simulink model "r2_deng_tvg_2013a"  (R2013a)
(part 3 of 43)

  edge_detect2/1(out) -> [mrst]  "mrst"
  edge_detect1/1(out) -> [msync]  "msync"
  edge_detect4/1(out) -> [clr_status]  "clr_status"
  Counter Free-Running/1 -> Relational Operator1/2, Relational Operator/2
  Constant1/1 -> Relational Operator/1
  Constant/1 -> Relational Operator1/1
  [local_time] -> slice1/1, slice2/1
  edge_detect3/1(out) -> [up_cnt_rst]  "mrst"
  Constant28/1 -> control/3(sim_3)
  Constant44/1 -> control/1(sim_1)
  Constant24/1 -> control/2(sim_2)
  Constant33/1 -> control/6(sim_6)
  Constant30/1 -> control/5(sim_5)
  Constant36/1 -> control/4(sim_4)
  Relational Operator/1 -> control/8(sim_8)
  Relational Operator1/1 -> control/7(sim_7)
  [tick_offset] -> ticks_since_mrst/3(offset)
  edge_detect10/1(out) -> [load_tick_offset]  "mrst"
  Constant20/1 -> control/9(sim_9)
  digitiser_id/1(in_digitiser_serial) -> bus_create/1(in1)
  digitiser_id/2(in_digitiser_type) -> bus_create/2(in2)
  Constant43/1 -> flag_setup/3(sim_3)
  Constant42/1 -> flag_setup/2(sim_2)
  Constant39/1 -> flag_setup/1(sim_1)
  Counter Free-Running3/1 -> Relational Operator4/2
  Constant48/1 -> Relational Operator4/1
  Relational Operator4/1 -> flag_setup/4(sim_4)
  Constant52/1 -> start_flag_msw/1(sim_1)
  Constant53/1 -> start_flag_lsw/1(sim_1)
  Constant51/1 -> end_flag_msw/1(sim_1)
  Constant50/1 -> end_flag_lsw/1(sim_1)
  Concat4/1 -> Delay49/1  "starttime"
  Concat5/1 -> Delay50/1  "stoptime"
  [flag_start_time] -> Delay46/1
  [local_time] -> Delay45/1, Delay47/1
  [flag_end_time] -> Delay48/1, Delay51/1
  Relational/1 -> Logical2/2  "start_okay"
  [flag_armed] -> Delay44/1
  Relational1/1 -> Logical4/2  "end_okay"
  Logical2/1 -> Delay23/1  "start_okay"
  Logical4/1 -> Logical3/1  "end_okay"
  edge_detect9/1(out) -> [load_flag_time]  "loadtimes"
  Constant4/1 -> Register1/1
  edge_detect8/1(out) -> [reset_flag_time]  "rst"
  [reset_flag_time] -> Register1/2
  [load_flag_time] -> Register1/3
  Register1/1 -> [flag_armed]  "armed"
  Relational Operator3/1 -> flag_setup/5(sim_5)
  Relational2/1 -> Delay22/1  "zero_stop"
  Constant2/1 -> Relational2/2
  Logical3/1 -> Logical1/2  "eokay"
  Counter Free-Running2/1 -> Relational Operator3/2
  Constant5/1 -> Relational Operator3/1
  Logical5/1 -> sample_masking/2(den_in)
  Constant49/1 -> start_time_msw/1(sim_1)
  Constant54/1 -> start_time_lsw/1(sim_1)
  Constant3/1 -> end_time_msw/1(sim_1)
  Constant11/1 -> end_time_lsw/1(sim_1)
  Relational3/1 -> Logical6/2  "start_okay"
  Relational4/1 -> Logical8/2  "end_okay"
  [start_time] -> Delay39/1
  Relational6/1 -> Delay15/1  "first_sample"
  [end_time] -> Delay41/1
  Relational7/1 -> Delay16/1  "last_sample"
  [sample_end] -> sample_masking/6(sample_end)
  [sample_start] -> sample_masking/5(sample_start)
  sample_masking/2(den_out) -> Delay126/1  "enable"
  sample_masking/3(data_mask) -> Delay127/1  "mask"
  edge_detect11/1(out) -> [reset_en_time]  "reset_en_time"
  Relational Operator5/1 -> control_output/2(sim_2)
  Counter Free-Running4/1 -> Relational Operator6/2, Relational Operator5/2
  Constant38/1 -> Relational Operator5/1
  edge_detect12/1(out) -> [load_en_time]  "load_en_time"
  Concat/1 -> Delay42/1
  Concat1/1 -> Delay43/1
  Constant22/1 -> Register2/1
  [reset_en_time] -> Register2/2
  [load_en_time] -> Register2/3
  Register2/1 -> [en_armed]  "armed"
  Logical6/1 -> Delay17/1  "start_okay"
  Logical8/1 -> Logical7/1  "end_okay"
  Logical7/1 -> Logical5/2
  Constant34/1 -> Delay37/1
  Relational5/1 -> Delay14/1
  Constant29/1 -> control_output/3(sim_3)
  Constant47/1 -> control_output/4(sim_4)
  Constant31/1 -> Relational Operator6/1
  Relational Operator6/1 -> control_output/1(sim_1)
  [data_enable] -> Delay129/1
  [sample_mask] -> Delay130/1
  Constant23/1 -> Mux3/2
  [adc_count] -> Concat3/1
  [adc_flag] -> Concat3/3
  [ndiode_flag] -> Concat3/4
  Constant55/1 -> Concat3/2
  Concat3/1 -> Mux3/3
  [flag_en] -> Mux3/1
  Constant46/1 -> tick_offset_msw/1(sim_1)
  Constant7/1 -> tick_offset_lsw/1(sim_1)
  Concat2/1 -> Register3/1
  [load_tick_offset] -> Register3/2
  Register3/1 -> [tick_offset]
  Delay1/1 -> [status0]
  fifo2/1(fifo_data80) -> pipeline104/1(d)  "data00"
  fifo2/2(fifo_dv) -> pipeline105/1(d)  "dv00"
  fifo2/3(word_start) -> pipeline106/1(d)  "ws00"
  fifo2/4(pkt_start) -> pipeline107/1(d)  "ps00"
  fifo2/5(fifo_full) -> Terminator3/1  "full00"
  fifo2/6(fifo_empty) -> Terminator6/1  "empty00"
  fifo3/1(fifo_data80) -> pipeline108/1(d)  "data01"
  fifo3/2(fifo_dv) -> pipeline109/1(d)  "dv01"
  fifo3/3(word_start) -> pipeline110/1(d)  "ws01"
  fifo3/4(pkt_start) -> pipeline111/1(d)  "ps01"
  pack_80_64_2/3(data64) -> pipeline123/1(d)  "d64_00"
  pack_80_64_2/2(valid64) -> pipeline122/1(d)  "v64_01"
  pack_80_64_2/1(ready64) -> pipeline121/1(d)  "r64_01"
  fifo3/5(fifo_full) -> Terminator4/1
  fifo3/6(fifo_empty) -> Terminator5/1
  [hdr_0x3101] -> bus_create3/1(in1)
  [pol1_id] -> bus_create3/2(in2)
  [hdr_0x3101] -> bus_create2/1(in1)
  [pol1_id] -> bus_create2/2(in2)
  [speadtime0] -> spead_pack2/4(hdr_heap_id), spead_pack2/8(hdr5_0x1600_DIR)  "timein0"
  bus_create3/1(bus_out) -> spead_pack2/9(hdr6_0x3101_DIR)
  [status2] -> spead_pack2/10(hdr7_0x3102_DIR)
  bus_create2/1(bus_out) -> spead_pack3/9(hdr6_0x3101_DIR)
  [status3] -> spead_pack3/10(hdr7_0x3102_DIR)
  [speadtime1] -> spead_pack3/8(hdr5_0x1600_DIR), spead_pack3/4(hdr_heap_id)  "timein1"
  pack_80_64_1/1(ready64) -> pipeline118/1(d)  "r64_00"
  pack_80_64_1/2(valid64) -> pipeline119/1(d)  "v64_00"
  pack_80_64_1/3(data64) -> pipeline120/1(d)  "d64_00"
  [spead_heapsize] -> spead_pack2/5(hdr_heap_size)
  [spead_heapoffset] -> spead_pack2/6(hdr_heap_offset)
  [spead_pktlen] -> spead_pack2/7(hdr_pkt_len_words)
  [spead_heapsize] -> spead_pack3/5(hdr_heap_size)
  [spead_heapoffset] -> spead_pack3/6(hdr_heap_offset)
  [spead_pktlen] -> spead_pack3/7(hdr_pkt_len_words)
  spead_pack3/4(data_overflow) -> Terminator2/1
  [adc_data_offset] -> spead_pack2/11(hdr8_0x3300)
  [adc_data_offset] -> spead_pack3/11(hdr8_0x3300)
  spead_pack2/4(data_overflow) -> Terminator1/1
  spead_pack2/3(eof) -> pipeline62/1(d)
  spead_pack2/1(data_out) -> pipeline60/1(d)  "packd"
  spead_pack2/2(valid_out) -> pipeline61/1(d)  "packv"
  spead_pack3/1(data_out) -> pipeline63/1(d)
  spead_pack3/2(valid_out) -> pipeline64/1(d)
  spead_pack3/3(eof) -> pipeline65/1(d)
  Inverter1/1 -> fifo3/2(fifo_we_en)
  [tvg_select1] -> Delay106/1
  Mux1/1 -> Assert1/1  "d80_0"
  [data_80_1] -> Delay109/1
  [tvg_pol1] -> Delay108/1
  Assert1/1 -> fifo3/1(data80), fifo2/1(data80)
  [fifoselect] -> Inverter1/1, fifo2/2(fifo_we_en)
  [gbe_txen] -> Logical13/1, Logical10/2
  Logical10/1 -> pipeline86/1(d)
  [gbe_port0] -> gbe0/5(tx_dest_port)
  Constant56/1 -> gbe0/8(rx_overrun_ack), gbe0/7(rx_ack)
  [spead_valid0] -> Logical10/1
  pipeline83/1(q) -> gbe0/2(tx_data)
  [gbe_ip0] -> gbe0/4(tx_dest_ip)
  [gbe_rst] -> pipeline68/1(d)
  [gbe_txen] -> Logical14/1, Logical9/2
  Logical9/1 -> pipeline85/1(d)
  [gbe_port1] -> gbe1/5(tx_dest_port)
  Constant18/1 -> gbe1/8(rx_overrun_ack), gbe1/7(rx_ack)
  [spead_valid1] -> Logical9/1
  pipeline80/1(q) -> gbe1/2(tx_data)
  [gbe_ip1] -> gbe1/4(tx_dest_ip)
  [gbe_rst] -> pipeline70/1(d)
  [gbe_txen] -> Logical15/1, Logical12/2
  Logical12/1 -> pipeline82/1(d)
  [gbe_port2] -> gbe2/5(tx_dest_port)
  Constant25/1 -> gbe2/8(rx_overrun_ack), gbe2/7(rx_ack)
  [spead_valid2] -> Logical12/1
  pipeline77/1(q) -> gbe2/2(tx_data)
  [gbe_ip2] -> gbe2/4(tx_dest_ip)
  [gbe_txen] -> Logical16/1, Logical11/2
  Logical11/1 -> pipeline75/1(d)
  [gbe_port3] -> gbe3/5(tx_dest_port)
  Constant21/1 -> gbe3/8(rx_overrun_ack), gbe3/7(rx_ack)
  [spead_data3] -> pipeline74/1(d)
  [gbe_ip3] -> gbe3/4(tx_dest_ip)
  [clr_status] -> pipeline69/1(d)
  [clr_status] -> pipeline71/1(d)
  [spead_eof0] -> Logical13/2
  [spead_eof1] -> Logical14/2
  Logical15/1 -> pipeline87/1(d)
  [spead_eof2] -> Logical15/2
  Logical16/1 -> pipeline76/1(d)
  [spead_eof3] -> Logical16/2
  gbe0/1(led_up) -> Terminator77/1
  gbe0/2(led_rx) -> Terminator67/1
  gbe0/3(led_tx) -> Terminator72/1
  gbe0/4(tx_afull) -> Terminator73/1
  gbe0/5(tx_overflow) -> Terminator75/1
  gbe0/6(rx_data) -> Terminator66/1
  gbe0/7(rx_valid) -> Terminator68/1
  gbe0/8(rx_source_ip) -> Terminator69/1
  gbe0/9(rx_source_port) -> Terminator70/1
  gbe0/10(rx_end_of_frame) -> Terminator71/1
  gbe0/11(rx_bad_frame) -> Terminator74/1
  gbe0/12(rx_overrun) -> Terminator76/1
  gbe1/1(led_up) -> Terminator13/1
  gbe1/2(led_rx) -> Terminator8/1
  gbe1/3(led_tx) -> Terminator40/1
  gbe1/4(tx_afull) -> Terminator43/1
  gbe1/5(tx_overflow) -> Terminator10/1
  gbe1/6(rx_data) -> Terminator7/1
  gbe1/7(rx_valid) -> Terminator9/1
  gbe1/8(rx_source_ip) -> Terminator34/1
  gbe1/9(rx_source_port) -> Terminator37/1
  gbe1/10(rx_end_of_frame) -> Terminator38/1
  gbe1/11(rx_bad_frame) -> Terminator46/1
  gbe1/12(rx_overrun) -> Terminator11/1
  gbe2/1(led_up) -> Terminator21/1
  gbe2/2(led_rx) -> Terminator22/1
  gbe2/3(led_tx) -> Terminator28/1
  gbe2/4(tx_afull) -> Terminator29/1
  gbe2/5(tx_overflow) -> Terminator17/1
  gbe2/6(rx_data) -> Terminator14/1
  gbe2/7(rx_valid) -> Terminator24/1
  gbe2/8(rx_source_ip) -> Terminator25/1
  gbe2/9(rx_source_port) -> Terminator26/1
  gbe2/10(rx_end_of_frame) -> Terminator27/1
  gbe2/11(rx_bad_frame) -> Terminator30/1
  gbe2/12(rx_overrun) -> Terminator19/1
  gbe3/1(led_up) -> Terminator35/1
  gbe3/2(led_rx) -> Terminator36/1
  gbe3/3(led_tx) -> Terminator45/1
  gbe3/4(tx_afull) -> Terminator47/1
  gbe3/5(tx_overflow) -> Terminator32/1
  gbe3/6(rx_data) -> Terminator31/1
  gbe3/7(rx_valid) -> Terminator39/1
  gbe3/8(rx_source_ip) -> Terminator41/1
  gbe3/9(rx_source_port) -> Terminator42/1
  gbe3/10(rx_end_of_frame) -> Terminator44/1
  gbe3/11(rx_bad_frame) -> Terminator48/1
  gbe3/12(rx_overrun) -> Terminator33/1
  Logical13/1 -> pipeline84/1(d)
  Logical14/1 -> pipeline81/1(d)
  [spead_data0] -> pipeline83/1(d)
  [spead_data1] -> pipeline80/1(d)
  [spead_data2] -> pipeline77/1(d)
  [spead_valid3] -> Logical11/1
  scale_wng0/1(in_reg) -> pipeline41/1(d)
  scale_wng1/1(in_reg) -> pipeline43/1(d)
  scale_wng_corr/1(in_reg) -> pipeline42/1(d)
  wng0/1(bus_out) -> pipeline78/1(d)
  wng1/1(bus_out) -> pipeline89/1(d)
  cwg0/1(bus_out) -> pipeline90/1(d)
  cwg_corr/1(bus_out) -> pipeline92/1(d), pipeline91/1(d)
  cwg1/1(bus_out) -> pipeline93/1(d)
  bus_addsub/1(dout) -> Delay105/1
  bus_addsub2/1(dout) -> Delay6/1
  bus_addsub3/1(dout) -> Delay9/1
  bus_addsub1/1(dout) -> Delay5/1
  bus_addsub4/1(dout) -> pipeline50/1(d)
  bus_mult/1(a*b) -> Scope4/3, bus_convert/1(din)
  bus_addsub5/1(dout) -> pipeline53/1(d)
  scale_out0/1(in_reg) -> pipeline51/1(d)
  scale_out1/1(in_reg) -> pipeline52/1(d)
  Constant35/1 -> scale_wng0/1(sim_1)
  Constant37/1 -> scale_wng1/1(sim_1)
  Constant57/1 -> scale_wng_corr/1(sim_1)
  Constant58/1 -> scale_cwg0/1(sim_1)
  scale_cwg0/1(in_reg) -> pipeline44/1(d)
  freq_cwg0/1(in_reg) -> pipeline45/1(d)
  Constant59/1 -> freq_cwg0/1(sim_1)
  Constant64/1 -> scale_out0/1(sim_1)
  Constant65/1 -> scale_out1/1(sim_1)
  Constant60/1 -> scale_cwg1/1(sim_1)
  scale_cwg1/1(in_reg) -> pipeline48/1(d)
  freq_cwg1/1(in_reg) -> pipeline49/1(d)
  Constant61/1 -> freq_cwg1/1(sim_1)
  Constant62/1 -> scale_cwg_corr/1(sim_1)
  scale_cwg_corr/1(in_reg) -> pipeline46/1(d)
  Constant63/1 -> freq_cwg_corr/1(sim_1)
  pipeline21/1(q) -> edge_detect12/1(in)
  pipeline22/1(q) -> edge_detect11/1(in)
  pipeline23/1(q) -> [sample_start]
  pipeline24/1(q) -> [sample_end]
  Delay42/1 -> [start_time]
  Delay43/1 -> [end_time]
  Delay49/1 -> [flag_start_time]
  Delay50/1 -> [flag_end_time]
  pipeline41/1(q) -> wng0/1(scale_16_14)
  pipeline42/1(q) -> wng_corr/1(scale_16_14)
  pipeline43/1(q) -> wng1/1(scale_16_14)
  pipeline44/1(q) -> cwg0/1(freq)
  pipeline45/1(q) -> cwg0/2(scale)
  pipeline46/1(q) -> cwg_corr/1(freq)
  pipeline48/1(q) -> cwg1/1(freq)
  pipeline49/1(q) -> cwg1/2(scale)
  pipeline10/1(q) -> [gbe_ip3]
  pipeline11/1(q) -> [gbe_ip2]
  pipeline13/1(q) -> [gbe_ip0]
  pipeline9/1(q) -> [gbe_port0]
  Delay102/1 -> Mux/1
  Delay103/1 -> Mux/2
  Delay104/1 -> Mux/3
  Delay106/1 -> Mux1/1
  Delay126/1 -> [data_enable]
  Delay127/1 -> [sample_mask]
  Delay128/1 -> tvg_spead_time_with_pkt_ctr/1(localtime64)
  Delay129/1 -> tvg_spead_time_with_pkt_ctr/2(data_enable)
  Delay130/1 -> tvg_spead_time_with_pkt_ctr/3(data_mask)
  Delay131/1 -> [tvg_ltime]
  Delay132/1 -> [tvg_stime]
  Delay133/1 -> [tvg_pol0]
  Delay134/1 -> [tvg_pol1]
  [tvg_pol0] -> Delay103/1
  [data_80_0] -> Delay104/1
  Delay109/1 -> Mux1/3
  Delay108/1 -> Mux1/2
  Delay105/1 -> Delay139/1
  Delay5/1 -> Delay7/1
  Delay6/1 -> Delay2/1
  Delay9/1 -> Delay8/1
  Delay139/1 -> Scope4/2, bus_addsub4/1(a)
  Delay7/1 -> bus_addsub5/1(a)
  Delay8/1 -> bus_addsub5/2(b), Scope3/1
  pipeline25/1(q) -> Concat/1
  pipeline26/1(q) -> Concat/2
  pipeline27/1(q) -> Concat1/1
  pipeline28/1(q) -> Concat1/2
  pipeline29/1(q) -> [hdr_0x3101]
  pipeline30/1(q) -> [pol0_id]
  pipeline31/1(q) -> [pol1_id]
  control/1(in_up_cnt_rst) -> pipeline/1(d)
  pipeline/1(q) -> edge_detect3/1(in)
  control/2(in_tvg_select0) -> pipeline1/1(d)
  control/3(in_tvg_select1) -> pipeline2/1(d)
  control/4(in_clr_status) -> pipeline3/1(d)
  control/5(in_gbe_rst) -> pipeline4/1(d)
  control/6(in_gbe_txen) -> pipeline5/1(d)
  control/7(in_msync) -> pipeline6/1(d)
  control/8(in_mrst) -> pipeline7/1(d)
  control/9(in_load_tick_offset) -> pipeline8/1(d)
  pipeline8/1(q) -> edge_detect10/1(in)
  pipeline7/1(q) -> edge_detect2/1(in)
  pipeline6/1(q) -> edge_detect1/1(in)
  pipeline5/1(q) -> [gbe_txen]
  pipeline4/1(q) -> [gbe_rst]
  pipeline3/1(q) -> edge_detect4/1(in)
  pipeline2/1(q) -> [tvg_select1]
  pipeline1/1(q) -> [tvg_select0]
  pipeline12/1(q) -> [gbe_ip1]
  pipeline16/1(q) -> pipeline124/1(d), pipeline125/1(d)
  pipeline14/1(q) -> [gbe_port1]
  gbe_iptx0/1(in_reg) -> pipeline13/1(d)
  gbe_iptx1/1(in_reg) -> pipeline12/1(d)
  gbe_iptx2/1(in_reg) -> pipeline11/1(d)
  gbe_iptx3/1(in_reg) -> pipeline10/1(d)
  tick_offset_msw/1(in_reg) -> pipeline17/1(d)
  pipeline17/1(q) -> Concat2/1
  tick_offset_lsw/1(in_reg) -> pipeline18/1(d)
  pipeline18/1(q) -> Concat2/2
  slice1/1 -> pipeline20/1(d)
  pipeline20/1(q) -> local_time_lsw/1(out_reg)
  slice2/1 -> pipeline19/1(d)
  pipeline19/1(q) -> local_time_msw/1(out_reg)
  end_time_lsw/1(in_reg) -> pipeline28/1(d)
  end_time_msw/1(in_reg) -> pipeline27/1(d)
  start_time_lsw/1(in_reg) -> pipeline26/1(d)
  start_time_msw/1(in_reg) -> pipeline25/1(d)
  control_output/4(in_sample_end) -> pipeline24/1(d)
  control_output/3(in_sample_start) -> pipeline23/1(d)
  control_output/2(in_reset_en_time) -> pipeline22/1(d)
  control_output/1(in_load_en_time) -> pipeline21/1(d)
  bus_create/1(bus_out) -> pipeline29/1(d)
  receptor_id/2(in_pol0_id) -> pipeline30/1(d)
  receptor_id/3(in_pol1_id) -> pipeline31/1(d)
  flag_setup/1(in_adc_count) -> pipeline32/1(d)
  flag_setup/2(in_adc_flag) -> pipeline33/1(d)
  flag_setup/3(in_ndiode_flag) -> pipeline34/1(d)
  flag_setup/4(in_load_flags) -> pipeline35/1(d)
  flag_setup/5(in_reset_flags) -> pipeline36/1(d)
  pipeline36/1(q) -> edge_detect8/1(in)
  pipeline35/1(q) -> edge_detect9/1(in)
  pipeline34/1(q) -> [ndiode_flag]
  pipeline33/1(q) -> [adc_flag]
  pipeline32/1(q) -> [adc_count]
  start_flag_msw/1(in_reg) -> pipeline37/1(d)
  pipeline37/1(q) -> Concat4/1
  start_flag_lsw/1(in_reg) -> pipeline38/1(d)
  pipeline38/1(q) -> Concat4/2
  end_flag_msw/1(in_reg) -> pipeline39/1(d)
  pipeline39/1(q) -> Concat5/1
  end_flag_lsw/1(in_reg) -> pipeline40/1(d)
  pipeline40/1(q) -> Concat5/2
  freq_cwg_corr/1(in_reg) -> pipeline47/1(d)
  pipeline47/1(q) -> cwg_corr/2(scale)
  pipeline53/1(q) -> Scope3/2, bus_mult1/1(a)
  pipeline52/1(q) -> bus_mult1/2(b)
  pipeline51/1(q) -> bus_mult/2(b)
  pipeline50/1(q) -> Scope4/1, bus_mult/1(a)
  pipeline54/1(q) -> [spead_data0]
  pipeline55/1(q) -> [spead_valid0]
  pipeline56/1(q) -> [spead_eof0]
  pipeline57/1(q) -> [spead_data1]
  pipeline58/1(q) -> [spead_valid1]
  pipeline59/1(q) -> [spead_eof1]
  pipeline60/1(q) -> [spead_data2]
  pipeline61/1(q) -> [spead_valid2]
  pipeline62/1(q) -> [spead_eof2]
  pipeline63/1(q) -> [spead_data3]
  pipeline64/1(q) -> [spead_valid3]
  pipeline65/1(q) -> [spead_eof3]
  [gbe_rst] -> pipeline66/1(d)
  pipeline66/1(q) -> gbe0/1(rst)
  [clr_status] -> pipeline67/1(d)
  pipeline67/1(q) -> gbe0/9(debug_rst)
  pipeline68/1(q) -> gbe1/1(rst)
  pipeline69/1(q) -> gbe1/9(debug_rst)
  pipeline70/1(q) -> gbe2/1(rst)
  pipeline71/1(q) -> gbe2/9(debug_rst)
  [gbe_rst] -> pipeline72/1(d)
  pipeline72/1(q) -> gbe3/1(rst)
  [clr_status] -> pipeline73/1(d)
  pipeline73/1(q) -> gbe3/9(debug_rst)
  pipeline86/1(q) -> gbe0/3(tx_valid)
  pipeline84/1(q) -> gbe0/6(tx_end_of_frame)
  pipeline85/1(q) -> gbe1/3(tx_valid)
  pipeline81/1(q) -> gbe1/6(tx_end_of_frame)
  pipeline82/1(q) -> gbe2/3(tx_valid)
  pipeline87/1(q) -> gbe2/6(tx_end_of_frame)
  pipeline74/1(q) -> gbe3/2(tx_data)
  pipeline75/1(q) -> gbe3/3(tx_valid)
  pipeline76/1(q) -> gbe3/6(tx_end_of_frame)
  pipeline78/1(q) -> Scope/1, bus_addsub/1(a)
  pipeline79/1(q) -> Scope/2, bus_addsub/2(b)
  pipeline88/1(q) -> Scope/3, bus_addsub1/1(a)
  wng_corr/1(bus_out) -> pipeline79/1(d), pipeline88/1(d)
  pipeline89/1(q) -> Scope/4, bus_addsub1/2(b)
  pipeline90/1(q) -> Scope/5, bus_addsub2/1(a)
  pipeline91/1(q) -> Scope/6, bus_addsub2/2(b)
  pipeline92/1(q) -> Scope/7, bus_addsub3/1(a)
  pipeline93/1(q) -> Scope/8, bus_addsub3/2(b)
  pipeline94/1(q) -> [data_80_0]
  pipeline95/1(q) -> [data_80_1]
  pipeline96/1(q) -> pack_80_64_00/1(data80)
  pipeline97/1(q) -> pack_80_64_00/2(valid80)
  pipeline98/1(q) -> pack_80_64_00/3(word_start)
  pipeline99/1(q) -> pack_80_64_00/4(pkt_start)
  pipeline100/1(q) -> pack_80_64_01/1(data80)
  pipeline101/1(q) -> pack_80_64_01/2(valid80)
  pipeline102/1(q) -> pack_80_64_01/3(word_start)
  pipeline103/1(q) -> pack_80_64_01/4(pkt_start)
  pipeline105/1(q) -> pack_80_64_1/2(valid80)
  pipeline104/1(q) -> pack_80_64_1/1(data80)
  pipeline106/1(q) -> pack_80_64_1/3(word_start)
  pipeline107/1(q) -> pack_80_64_1/4(pkt_start)
  pipeline108/1(q) -> pack_80_64_2/1(data80)
  pipeline109/1(q) -> pack_80_64_2/2(valid80)
  pipeline110/1(q) -> pack_80_64_2/3(word_start)
  pipeline111/1(q) -> pack_80_64_2/4(pkt_start)
  pipeline112/1(q) -> spead_pack0/1(data64_ready)
  pipeline113/1(q) -> spead_pack0/2(data64_valid)
  pipeline114/1(q) -> spead_pack0/3(data64)
  pipeline115/1(q) -> spead_pack1/1(data64_ready)
  pipeline116/1(q) -> spead_pack1/2(data64_valid)
  pipeline117/1(q) -> spead_pack1/3(data64)
  pipeline118/1(q) -> spead_pack2/1(data64_ready)
  pipeline119/1(q) -> spead_pack2/2(data64_valid)
  pipeline120/1(q) -> spead_pack2/3(data64)
  pipeline121/1(q) -> spead_pack3/1(data64_ready)
  pipeline122/1(q) -> spead_pack3/2(data64_valid)
  pipeline123/1(q) -> spead_pack3/3(data64)
  pipeline125/1(q) -> [gbe_port2]
  pipeline124/1(q) -> [gbe_port3]
  pipeline15/1(q) -> pipeline14/1(d), pipeline9/1(d)
  Delay2/1 -> bus_addsub4/2(b)
  Delay12/1 -> [status3]
  Delay11/1 -> [status2]
  Delay10/1 -> [status1]
  Delay13/1 -> Logical8/1, Logical6/1
  Delay14/1 -> Logical7/2
  Delay15/1 -> Delay18/1
  Delay16/1 -> Delay19/1
  Delay17/1 -> Logical5/1
  Delay18/1 -> Delay20/1
  Delay19/1 -> Delay21/1
  Delay20/1 -> sample_masking/3(first_samples)
  Delay21/1 -> sample_masking/4(last_samples)
  Delay22/1 -> Logical3/2
  Delay23/1 -> Logical1/1
  Delay24/1 -> Delay25/1
  Delay25/1 -> Delay26/1
  Delay26/1 -> Delay27/1
  Delay27/1 -> sample_masking/1(timei)
  sample_masking/4(flag_valid) -> Delay28/1
  Delay28/1 -> [flag_en]
  Logical1/1 -> sample_masking/7(flag_en)  "flag_en"
  sample_masking/1(timeo) -> Delay29/1
  Delay29/1 -> [masked_time]
  [local_time] -> Delay30/1
  [en_armed] -> Delay31/1
  [local_time] -> Delay32/1, Delay34/1, Delay38/1, Delay40/1
  [start_time] -> Delay33/1
  [end_time] -> Delay35/1, Delay36/1
  Delay30/1 -> Delay24/1
  Delay31/1 -> Delay13/1
  Delay32/1 -> Relational3/1
  Delay33/1 -> Relational3/2
  Delay34/1 -> Relational4/1
  Delay35/1 -> Relational4/2
  Delay36/1 -> Relational5/1
  Delay37/1 -> Relational5/2
  Delay38/1 -> Relational6/1
  Delay39/1 -> Relational6/2
  Delay40/1 -> Relational7/1
  Delay41/1 -> Relational7/2
  Delay44/1 -> Logical4/1, Logical2/1
  Delay45/1 -> Relational/1
  Delay46/1 -> Relational/2
  Delay47/1 -> Relational1/1
  Delay48/1 -> Relational1/2
  Delay51/1 -> Relational2/1
  bus_convert/1(dout) -> Scope1/1, pipeline94/1(d)
  bus_expand3/1(msb_out8) -> d80_snap0/1(in_s0)
  bus_expand3/2(out7) -> d80_snap0/2(in_s1)
  bus_expand3/3(out6) -> d80_snap0/3(in_s2)
  bus_expand3/4(out5) -> d80_snap0/4(in_s3)
  bus_expand3/5(out4) -> d80_snap0/5(in_s4)
  bus_expand3/6(out3) -> d80_snap0/6(in_s5)
  bus_expand3/7(out2) -> d80_snap0/7(in_s6)
  bus_expand3/8(lsb_out1) -> d80_snap0/8(in_s7)
  Constant32/1 -> d80_snap0/10(trig)
  [data_80_0] -> bus_expand3/1(bus_in)
  Constant41/1 -> d80_snap0/9(we)
  bus_expand1/4(out5) -> fifo_snap0/4(in_s3)
  bus_expand1/5(out4) -> fifo_snap0/5(in_s4)
  bus_expand1/6(out3) -> fifo_snap0/6(in_s5)
  bus_expand1/7(out2) -> fifo_snap0/7(in_s6)
  bus_expand1/8(lsb_out1) -> fifo_snap0/8(in_s7)
  Constant40/1 -> fifo_snap0/10(trig)
  [fifo80_0] -> bus_expand1/1(bus_in)
  Assert2/1 -> fifo_snap0/9(we)
  bus_expand1/3(out6) -> fifo_snap0/3(in_s2)
  bus_expand1/2(out7) -> fifo_snap0/2(in_s1)
  bus_expand1/1(msb_out8) -> fifo_snap0/1(in_s0)
  fifo0/2(fifo_dv) -> [fifo_dv0], pipeline97/1(d)  "dv00"
  bus_expand2/4(out5) -> d80_snap1/4(in_s3)
  bus_expand2/5(out4) -> d80_snap1/5(in_s4)
  bus_expand2/6(out3) -> d80_snap1/6(in_s5)
  bus_expand2/7(out2) -> d80_snap1/7(in_s6)
  bus_expand2/8(lsb_out1) -> d80_snap1/8(in_s7)
  [data_80_1] -> bus_expand2/1(bus_in)
  Constant67/1 -> d80_snap1/9(we)
  bus_expand2/3(out6) -> d80_snap1/3(in_s2)
  bus_expand2/2(out7) -> d80_snap1/2(in_s1)
  bus_expand2/1(msb_out8) -> d80_snap1/1(in_s0)
  Constant68/1 -> d80_snap1/10(trig)
  bus_expand4/4(out5) -> fifo_snap1/4(in_s3)
  bus_expand4/5(out4) -> fifo_snap1/5(in_s4)
  bus_expand4/6(out3) -> fifo_snap1/6(in_s5)
  bus_expand4/7(out2) -> fifo_snap1/7(in_s6)
  bus_expand4/8(lsb_out1) -> fifo_snap1/8(in_s7)
  Constant69/1 -> fifo_snap1/10(trig)
  [fifo80_1] -> bus_expand4/1(bus_in)
  Assert3/1 -> fifo_snap1/9(we)
  bus_expand4/3(out6) -> fifo_snap1/3(in_s2)
  bus_expand4/2(out7) -> fifo_snap1/2(in_s1)
  bus_expand4/1(msb_out8) -> fifo_snap1/1(in_s0)
  [fifo_dv0] -> Assert2/1
  [fifo_dv1] -> Assert3/1
  bus_convert1/1(dout) -> Scope2/1, pipeline95/1(d)
  bus_mult1/1(a*b) -> Scope3/3, bus_convert1/1(din)
